simulink library "LibraryModel"  (R2016b)
settings: Solver=VariableStepAuto  StartTime=0.0  StopTime=10.0  RelTol=1e-3
libraries: LibraryArchitecture x3
settings Model: Creator=Nathan  LastModifiedBy=Nathan

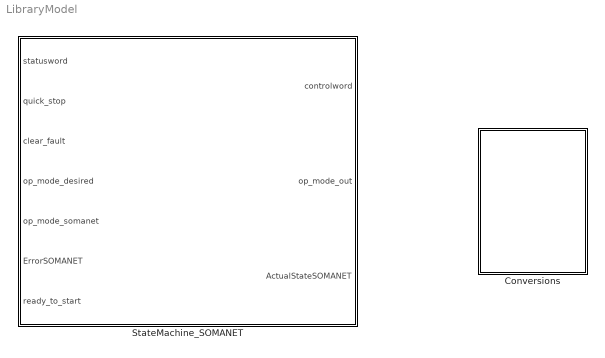
== system LibraryModel ==
  Conversions : Subsystem
  StateMachine_SOMANET : Stateflow chart  TreatAsAtomicUnit=on

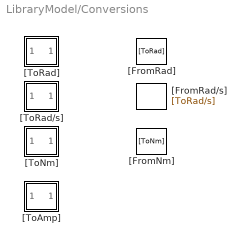
== system LibraryModel/Conversions ==
  "[FromNm]" : LibraryArchitecture/Conversions/[ToNm]
  "[FromRad/s]" : LibraryArchitecture/Conversions/[ToRad//s]
  "[FromRad]" : LibraryArchitecture/Conversions/[ToRad]
  "[ToAmp]" : Subsystem
  "[ToNm]" : Subsystem
  "[ToRad/s]" : Subsystem
  "[ToRad]" : Subsystem

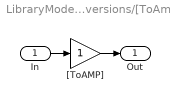
== system LibraryModel/Conversions/[ToAmp] ==
  In : Inport
  "[ToAMP]" : Gain
  Out : Outport
  wires:
  "[ToAMP]"/1 -> Out/1
  In/1 -> "[ToAMP]"/1

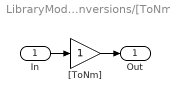
== system LibraryModel/Conversions/[ToNm] ==
  In : Inport
  "[ToNm]" : Gain
  Out : Outport
  wires:
  In/1 -> "[ToNm]"/1
  "[ToNm]"/1 -> Out/1

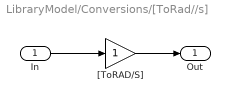
== system LibraryModel/Conversions/[ToRad//s] ==
  In : Inport
  "[ToRAD/S]" : Gain
  Out : Outport
  wires:
  In/1 -> "[ToRAD/S]"/1
  "[ToRAD/S]"/1 -> Out/1

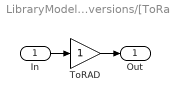
== system LibraryModel/Conversions/[ToRad] ==
  In : Inport
  ToRAD : Gain
  Out : Outport
  wires:
  ToRAD/1 -> Out/1
  In/1 -> ToRAD/1

== stateflow chart LibraryModel/StateMachine_SOMANET ==
  data: statusword input uint16; controlword output double; quick_stop input boolean; clear_fault input; op_mode_desired input int8; op_mode_somanet input; op_mode_out output int8; ActualStateSOMANET output; ErrorSOMANET input; ready_to_start input
